simulink model "sim_vsc"  (R2022a)
settings: Solver=ode45  StartTime=0.0  StopTime=Tfin  FixedStep=1e-3  MaxStep=1e-2  MinStep=1e-3  RelTol=5e-3
undefined symbols (not defined in the file or in its folder): c_ref, csi, KM, psir, refPoses, Ts, ze0
libraries: slpidlib x1, simulink x1
settings Model: PacingRate=0.750000  Creator=The MathWorks, Inc.  LastModifiedBy=vin
settings SolverCC: ZeroCrossAlgorithm=Adaptive  AlgebraicLoopSolver=TrustRegion  DecoupledContinuousIntegration=on  MinimalZcImpactIntegration=on
settings DataIOCC: SaveOutput=off  SignalLogging=off  DSMLogging=off  SaveTime=off  ReturnWorkspaceOutputs=off
settings DebuggingCC: UnconnectedInputMsg=warning  UnconnectedOutputMsg=warning  UnconnectedLineMsg=warning  SFMachineParentedDataDiag=warning  ArithmeticOperatorsInVariantConditions=warning
settings ModelReferenceCC: PropagateSignalLabelsOutOfModel=off
settings SFSimCC: SimUseLocalCustomCode=off  CustomCodeUndefinedFunction=UseInterfaceOnly
settings RTWCC: RTWUseLocalCustomCode=off  DLArmComputeVersion=19.05

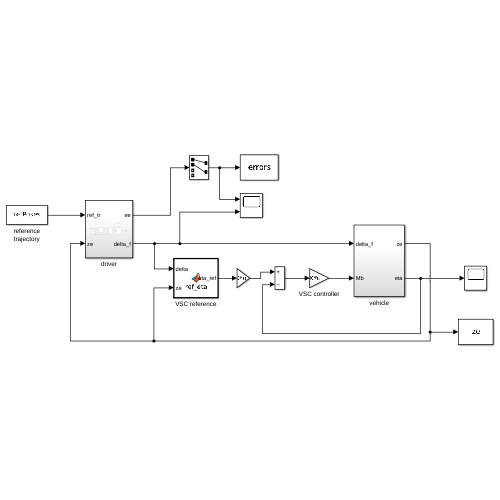
[thumbnail: Simulink's stored preview of the top-level diagram]
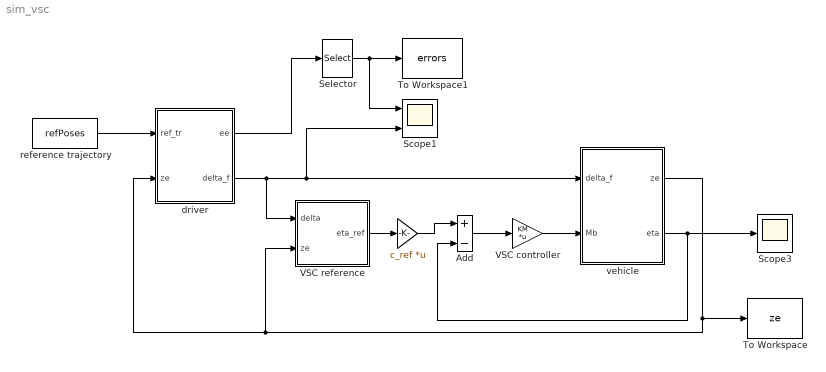
== system sim_vsc ==
  " " : Gain  Gain=c_ref  Multiplication=Matrix(K*u)
  Add : Sum  Inputs=+-
  Scope1 : Scope  NumInputPorts=2
  Scope3 : Scope
  Selector : Selector  InputPortWidth=4  IndexOptions=Index vector (dialog)  Indices=1:2  OutputSizes=1
  To Workspace : ToWorkspace  VariableName=ze  SaveFormat=Timeseries  SampleTime=-1
  To Workspace1 : ToWorkspace  VariableName=errors  SaveFormat=Timeseries  SampleTime=-1
  VSC controller : Gain  Gain=KM  Multiplication=Matrix(K*u)
  VSC reference : MATLAB Function  TreatAsAtomicUnit=on
  driver : Subsystem
  reference trajectory : Constant  Value=refPoses
  vehicle : Subsystem
  wires:
  Selector/1 -> To Workspace1/1, Scope1/1
  vehicle/1(ze) -> VSC reference/2(ze), driver/2(ze), To Workspace/1
  driver/2(delta_f) -> VSC reference/1(delta), vehicle/1(delta_f), Scope1/2
  reference trajectory/1 -> driver/1(ref_tr)
  driver/1(ee) -> Selector/1
  Add/1 -> VSC controller/1
  vehicle/2(eta) -> Scope3/1, Add/2
  VSC controller/1 -> vehicle/2(Mb)
  VSC reference/1(eta_ref) -> " "/1
  " "/1 -> Add/1

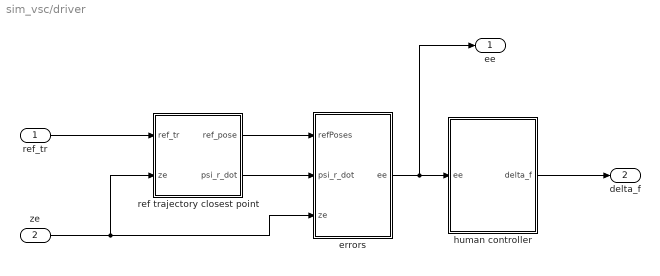
== system sim_vsc/driver ==
  ref_tr : Inport
  ze : Inport  Port=2
  errors : Subsystem
  human controller : Subsystem
  ref trajectory closest point : Subsystem
  ee : Outport
  delta_f : Outport  Port=2
  wires:
  ref trajectory closest point/1(ref_pose) -> errors/1(refPoses)
  ref trajectory closest point/2(psi_r_dot) -> errors/2(psi_r_dot)
  human controller/1(delta_f) -> delta_f/1
  ref_tr/1 -> ref trajectory closest point/1(ref_tr)
  errors/1(ee) -> ee/1, human controller/1(ee)
  ze/1 -> ref trajectory closest point/2(ze), errors/3(ze)

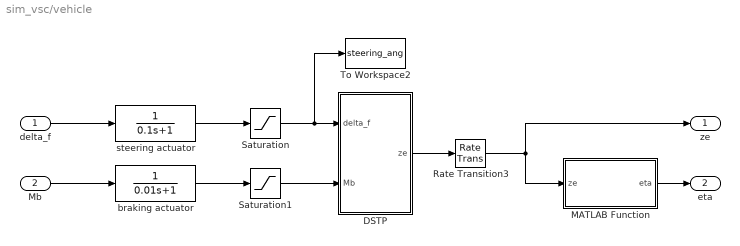
== system sim_vsc/vehicle ==
  delta_f : Inport
  Mb : Inport  Port=2
  " braking actuator" : TransferFcn  Denominator=[0.01 1]
  DSTP : Subsystem
  MATLAB Function : MATLAB Function  TreatAsAtomicUnit=on
  Rate Transition3 : RateTransition  InitialCondition=ze0  OutPortSampleTime=Ts
  Saturation : Saturate  UpperLimit=0.6  LowerLimit=-0.6
  Saturation1 : Saturate  UpperLimit=6.5e4  LowerLimit=-6.5e4
  To Workspace2 : ToWorkspace  VariableName=steering_ang  SaveFormat=Timeseries  SampleTime=-1
  steering actuator : TransferFcn  Denominator=[0.1 1]
  ze : Outport  VectorParamsAs1DForOutWhenUnconnected=off
  eta : Outport  Port=2  VectorParamsAs1DForOutWhenUnconnected=off
  wires:
  DSTP/1(ze) -> Rate Transition3/1
  Rate Transition3/1 -> ze/1, MATLAB Function/1(ze)
  delta_f/1 -> steering actuator/1
  steering actuator/1 -> Saturation/1
  Mb/1 -> " braking actuator"/1
  Saturation/1 -> To Workspace2/1, DSTP/1(delta_f)
  " braking actuator"/1 -> Saturation1/1
  Saturation1/1 -> DSTP/2(Mb)
  MATLAB Function/1(eta) -> eta/1

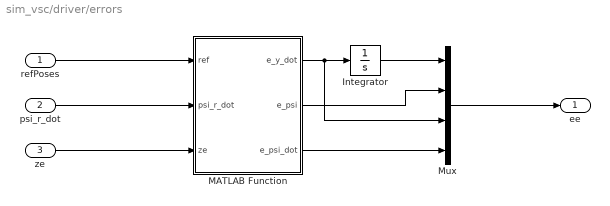
== system sim_vsc/driver/errors ==
  refPoses : Inport
  psi_r_dot : Inport  Port=2
  ze : Inport  Port=3
  Integrator : Integrator
  MATLAB Function : MATLAB Function  TreatAsAtomicUnit=on
  Mux : Mux
  ee : Outport
  wires:
  Integrator/1 -> Mux/1
  MATLAB Function/2(e_psi) -> Mux/2
  MATLAB Function/3(e_psi_dot) -> Mux/4
  MATLAB Function/1(e_y_dot) -> Mux/3, Integrator/1
  Mux/1 -> ee/1
  psi_r_dot/1 -> MATLAB Function/2(psi_r_dot)
  ze/1 -> MATLAB Function/3(ze)
  refPoses/1 -> MATLAB Function/1(ref)

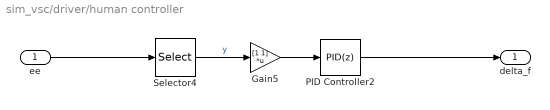
== system sim_vsc/driver/human controller ==
  ee : Inport
  Gain5 : Gain  Gain=[1 1]  Multiplication=Matrix(K*u)
  PID Controller2 : slpidlib/PID Controller  Controller=PID  Form=Parallel  TimeDomain=Discrete-time  UseExternalTs=off  SampleTime=0.05  IntegratorMethod=Forward Euler  FilterMethod=Forward Euler  ControllerParametersSource=internal  P=-0.0720009817402732  I=-0.00360229941130217  UseKiTs=off  D=-0.318956094963778  N=38.4333791808338  UseFilter=on  TunerSelectOption=Transfer Function Based (PID Tuner App)  InitialConditionSource=internal  InitialConditionForIntegrator=0  InitialConditionForFilter=0  DifferentiatorICPrevScaledInput=0  ExternalReset=none  TrackingMode=off  Kt=1  LimitOutput=off  SatLimitsSource=internal  UpperSaturationLimit=inf  LowerSaturationLimit=-inf  LinearizeAsGain=on  AntiWindupMode=none  Kb=1  POutMin=[]  POutMax=[]  IOutMin=[]  IOutMax=[]  DOutMin=[]  DOutMax=[]  NOutMin=[]  NOutMax=[]  SumOutMin=[]  SumOutMax=[]  SaturationOutMin=[]  SaturationOutMax=[]  PParamMin=[]  PParamMax=[]  IParamMin=[]  IParamMax=[]  DParamMin=[]  DParamMax=[]  NParamMin=[]  NParamMax=[]  KbParamMin=[]  KbParamMax=[]  KtParamMin=[]  KtParamMax=[]  KbOutMin=[]  KbOutMax=[]  KtOutMin=[]  KtOutMax=[]  IntegratorOutMin=[]  IntegratorOutMax=[]  FilterOutMin=[]  FilterOutMax=[]  SumI1OutMin=[]  SumI1OutMax=[]  SumI2OutMin=[]  SumI2OutMax=[]  SumI3OutMin=[]  SumI3OutMax=[]  SumI4OutMin=[]  SumI4OutMax=[]  SumDOutMin=[]  SumDOutMax=[]  DifferentiatorOutMin=[]  DifferentiatorOutMax=[]  FilterDiffOutCoefMin=[]  FilterDiffOutCoefMax=[]  ReciprocalOutMin=[]  ReciprocalOutMax=[]  SumDenOutMin=[]  SumDenOutMax=[]  SumNumOutMin=[]  SumNumOutMax=[]  DivideOutMin=[]  DivideOutMax=[]  UdiffTsProdOutMin=[]  UdiffTsProdOutMax=[]  NTsProdOutMin=[]  NTsProdOutMax=[]  UintegralTsProdOutMin=[]  UintegralTsProdOutMax=[]  UngainTsProdOutMin=[]  UngainTsProdOutMax=[]  ClampingZeroOutDataTypeStr=Inherit: Inherit via back propagation  ClampingZeroOutMin=[]  ClampingZeroOutMax=[]  FilterDenConstantOutDataTypeStr=Inherit: Inherit via back propagation  FilterDenConstantOutMin=[]  FilterDenConstantOutMax=[]  PCopyOutDataTypeStr=Inherit: Inherit via back propagation  PCopyOutMin=[]  PCopyOutMax=[]  NCopyOutDataTypeStr=Inherit: Inherit via back propagation  NCopyOutMin=[]  NCopyOutMax=[]  IntegratorContinuousStateAttributes=''  IntegratorStateMustResolveToSignalObject=off  IntegratorRTWStateStorageClass=Auto  FilterContinuousStateAttributes=''  FilterStateMustResolveToSignalObject=off  FilterRTWStateStorageClass=Auto  ParallelPVariant=InternalParameters  IdealPVariant=Disabled  IVariant=InternalParameters  DVariant=InternalParameters  IntegratorVariant=Discrete  SatVariant=Disabled  AWVariant=Passthrough  PCopyVariant=Disabled  TRVariant=Disabled  FdbkBlocksVariant=Forward  IdealPFdbkVariant=Disabled  SatFdbkVariant=Disabled  DerivativeFilterVariant=ForwardEulerFilter  NVariant=InternalParameters  NCopyVariant=Disabled  FilterICVariant=InternalICsFilter  IntegratorICVariant=InternalICs  ExternalResetVariant=Disabled  TRSumVariant=Passthrough  SumFdbkVariant=Disabled  SumVariant=Sum_PID  TsampFilterVariant=InternalTs  TsampNgainVariant=Passthrough  TsampIntegralVariant=Passthrough  ExternalSaturationOutDataTypeStr=Inherit: Same as second input  aMode=0
  Selector4 : Selector  InputPortWidth=4  IndexOptions=Index vector (dialog)  Indices=1:2  OutputSizes=1
  delta_f : Outport
  wires:
  ee/1 -> Selector4/1
  Gain5/1 -> PID Controller2/1
  Selector4/1 -> Gain5/1  "y"
  PID Controller2/1 -> delta_f/1

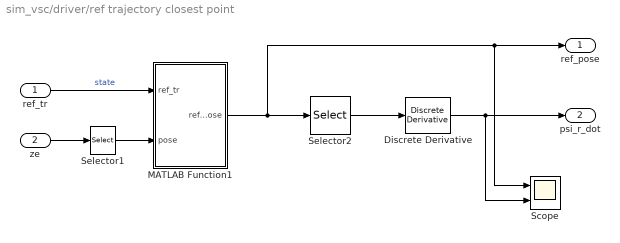
== system sim_vsc/driver/ref trajectory closest point ==
  ref_tr : Inport
  ze : Inport  Port=2
  Discrete Derivative : simulink/Discrete/Discrete Derivative  gainval=1  ICPrevScaledInput=psir(1)/Ts  OutMin=[]  OutMax=[]  OutDataType=fixdt(1, 16)  OutScaling=2^-10  DoSatur=off
  MATLAB Function1 : MATLAB Function  TreatAsAtomicUnit=on
  Scope : Scope  NumInputPorts=2
  Selector1 : Selector  InputPortWidth=6  IndexOptions=Index vector (dialog)  Indices=1:3  OutputSizes=1
  Selector2 : Selector  InputPortWidth=3  IndexOptions=Index vector (dialog)  Indices=3  OutputSizes=1
  ref_pose : Outport
  psi_r_dot : Outport  Port=2
  wires:
  ze/1 -> Selector1/1
  Selector1/1 -> MATLAB Function1/2(pose)
  ref_tr/1 -> MATLAB Function1/1(ref_tr)  "state"
  Selector2/1 -> Discrete Derivative/1
  MATLAB Function1/1(ref_pose) -> Scope/1, ref_pose/1, Selector2/1
  Discrete Derivative/1 -> Scope/2, psi_r_dot/1

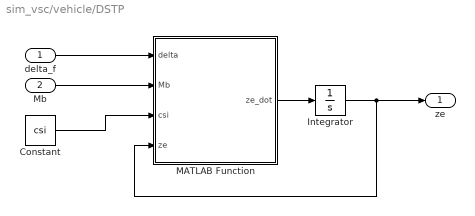
== system sim_vsc/vehicle/DSTP ==
  delta_f : Inport
  Mb : Inport  Port=2
  Constant : Constant  Value=csi
  Integrator : Integrator  InitialCondition=ze0
  MATLAB Function : MATLAB Function  TreatAsAtomicUnit=on
  ze : Outport
  wires:
  Integrator/1 -> ze/1, MATLAB Function/4(ze)
  delta_f/1 -> MATLAB Function/1(delta)
  MATLAB Function/1(ze_dot) -> Integrator/1
  Mb/1 -> MATLAB Function/2(Mb)
  Constant/1 -> MATLAB Function/3(csi)

== matlab function sim_vsc/VSC reference ==
  data: delta input; ze input; eta_ref output
function eta_ref=ref_eta(delta,ze) 

% Parameters
lf=1.2;     % m
lr=1.6;     % m
l=lr+lf;    % m
m=1575;     % kg
J=4000;     % kg*m^2
cf=27e3;    % N/rad
cr=20e3;    % N/rad
c1=-2*(cf+cr);
c2=-2*(cf*lf-cr*lr);
c3=-2*(cf*lf^2+cr*lr^2);

% Long. speed
vx=ze(4);

% Model matrices
Aeta=[c1/m/vx -1+c2/m/vx^2; c2/J c3/J/vx];
Bs=[2*cf/m/vx;2*cf*lf/J];

% Reference vector
eta_ref=-inv(Aeta)*Bs*delta;

% To improve the numerical efficiency, the inverse matrix can be 
% computed off-line analytically and directly implemented here.

== matlab function sim_vsc/driver/errors/MATLAB Function ==
  data: e_y_dot output; ref input; psi_r_dot input; e_psi output; e_psi_dot output; ze input
function [e_y_dot,e_psi,e_psi_dot]=errors(ref,psi_r_dot,ze)

e_psi=ze(3)-ref(3);
e_psi_dot=ze(6)-psi_r_dot;
e_y_dot=ze(5)+ze(4)*e_psi;

== matlab function sim_vsc/driver/ref trajectory closest point/MATLAB Function1 ==
  data: ref_tr input; ref_pose output; pose input
function ref_pose=ref_gen(ref_tr,pose)

N=size(ref_tr,1);

% point of the reference trajectory closest to the vehicle
dis=vecnorm(ref_tr(:,1:2)'-pose(1:2)*ones(1,N));
[~,im]=min(dis);
ref_pose=ref_tr(im,:)';

== matlab function sim_vsc/vehicle/MATLAB Function ==
  data: ze input; eta output
function eta=DSTbeta_states(ze)

beta=atan2(ze(5),ze(4));

eta=[beta;ze(6)];

== matlab function sim_vsc/vehicle/DSTP/MATLAB Function ==
  data: delta input; Mb input; csi input; ze input; ze_dot output
function ze_dot=single_track_model(delta,Mb,csi,ze) 

% Parameters
lf=1.2;     % m
lr=1.6;     % m
m=1575;     % kg
J=4000;     % kg*m^2
cf=27e3;    % N/rad
cr=20e3;    % N/rad

% State variables
X=ze(1);
Y=ze(2);
psi=ze(3);
vx=ze(4);
vy=ze(5);
w=ze(6);

% Slip angles
betaf=atan2(vy+lf*w,vx)-delta;
betar=atan2(vy-lr*w,vx);
%beta=atan2(vy,vx);

% Forces
Fyf=-pacejka_mf(betaf,cf,m,csi)*cos(delta);
Fyr=-pacejka_mf(betar,cr,m,csi);

% State equations
X_dot=vx*cos(psi)-vy*sin(psi);
Y_dot=vx*sin(psi)+vy*cos(psi);
psi_dot=w;
vx_dot=0;
vy_dot=-vx*w+2/m*(Fyf+Fyr);
w_dot=2/J*(lf*Fyf-lr*Fyr)+Mb/J;

% State derivative
ze_dot=[X_dot;Y_dot;psi_dot;vx_dot;vy_dot;w_dot];

end

function F=pacejka_mf(beta,c,m,csi)

Fz=m/4*9.81;
p=zeros(1,4);
p(1)=Fz*csi;          
p(2)=1.5;
p(3)=c/p(1)/p(2);   
p(4)=-0.5;

F=p(1)*sin(p(2)*atan(p(3)*beta-p(4)*(p(3)*beta-atan(p(3)*beta))));

end
